simulink model "SurfaceVesselModel"  (R2024a)
settings: Solver=VariableStepAuto  StartTime=0.0  StopTime=10.0  RelTol=1e-3
values from neighbouring files (symbols this model uses):
  B = [1 1; 0 0; d/2 -d/2]    [init.m]
  D = [   4.3411      0       0 ... (first row only)    [init.m]
  M = [   26.4272    0           0 ... (first row only)    [init.m]
libraries: SignalEditorBlockLib x1
settings Model: Creator=berto  LastModifiedBy=berto

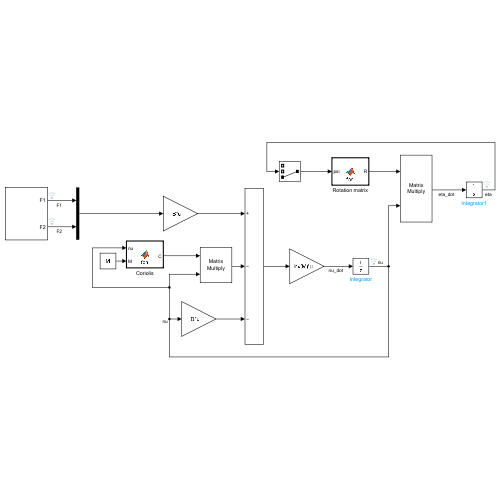
[thumbnail: Simulink's stored preview of the top-level diagram]
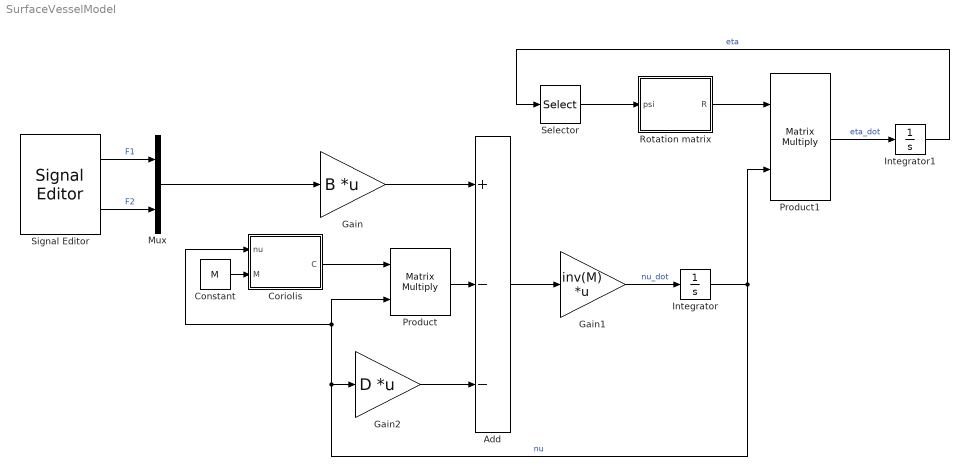
== system SurfaceVesselModel ==
  Add : Sum  Inputs=+--
  Constant : Constant  Value=M
  Coriolis : MATLAB Function  TreatAsAtomicUnit=on
  Gain : Gain  Gain=B  Multiplication=Matrix(K*u)
  Gain1 : Gain  Gain=inv(M)  Multiplication=Matrix(K*u)
  Gain2 : Gain  Gain=D  Multiplication=Matrix(K*u)
  Integrator : Integrator
  Integrator1 : Integrator
  Mux : Mux  Inputs=2
  Product : Product  Multiplication=Matrix(*)
  Product1 : Product  Multiplication=Matrix(*)
  Rotation matrix : MATLAB Function  TreatAsAtomicUnit=on
  Selector : Selector  InputPortWidth=3  IndexOptions=Index vector (dialog)  Indices=3  OutputSizes=1
  Signal Editor : SignalEditorBlockLib/Signal Editor  FileName=ControlSignals.mat  ActiveScenario=Test1  ActiveSignal=F1  IsBus=off  OutputBusObjectStr=Bus: BusObject  SampleTime=0.1  ZeroCross=off  OutputAfterFinalValue=Setting to zero  Unit=inherit  PreserveSignalName=on  ApplySigPropsToAllScenarios=on  ApplySigPropsToAllSignals=off
  wires:
  Signal Editor/1 -> Mux/1  "F1"
  Signal Editor/2 -> Mux/2  "F2"
  Mux/1 -> Gain/1
  Integrator/1 -> Coriolis/1(nu), Product/2, Gain2/1, Product1/2  "nu"
  Gain1/1 -> Integrator/1  "nu_dot"
  Gain/1 -> Add/1
  Add/1 -> Gain1/1
  Gain2/1 -> Add/3
  Product/1 -> Add/2
  Coriolis/1(C) -> Product/1
  Constant/1 -> Coriolis/2(M)
  Rotation matrix/1(R) -> Product1/1
  Product1/1 -> Integrator1/1  "eta_dot"
  Integrator1/1 -> Selector/1  "eta"
  Selector/1 -> Rotation matrix/1(psi)

== matlab function SurfaceVesselModel/Rotation matrix ==
  data: psi input; R output
function R = fcn(psi)

% Calculate R
R = [cos(psi), -sin(psi), 0; sin(psi), cos(psi), 0; 0, 0, 1];

== matlab function SurfaceVesselModel/Coriolis ==
  data: nu input; C output; M input
function C = fcn(nu, M)

% Get u, v, r from nu
u = nu(1);
v = nu(2);
r = nu(3);

% Calculate C
C = [0, 0, -M(2,2)*v - M(2,3)*r;
     0, M(1,1)*u, 0;
     M(2,2)*v + M(2,3)*r, -M(1,1)*u, 0];
